simulink model "CANRXcommunication"  (R2024a)
settings: Solver=VariableStepAuto  StartTime=0.0  StopTime=10.0  RelTol=1e-3
undefined symbols (not defined in the file or in its folder): canChannel
libraries: canlib x2, canmsglib x1
settings Model: DataDictionary=BMS_System_dict1.sldd  Creator=hirah  LastModifiedBy=hirah

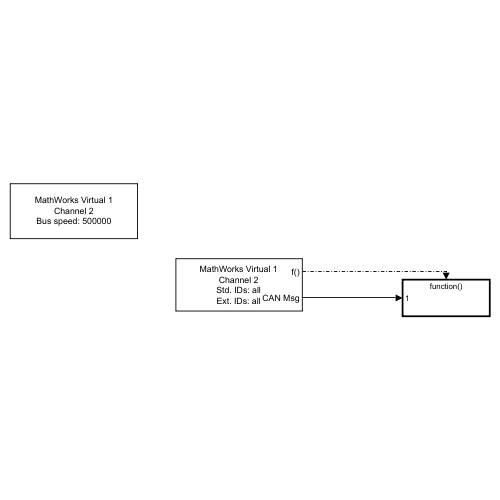
[thumbnail: Simulink's stored preview of the top-level diagram]
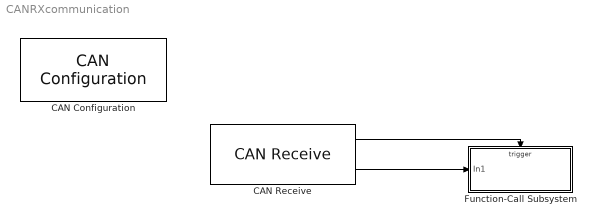
== system CANRXcommunication ==
  CAN Configuration : canlib/CAN Configuration  BlockHandle=570.0001  Device=MathWorks Virtual 1 (Channel 2)  DeviceMenu=MathWorks Virtual 1 (Channel 2)  ObjConstructor=canChannel('MathWorks', 'Virtual 1', 2)  BusSpeed=500000  EnableBitParameters=off  AckMode=Normal
  CAN Receive : canlib/CAN Receive  BlockHandle=729.0002  Device=MathWorks Virtual 1 (Channel 2)  DeviceMenu=MathWorks Virtual 1 (Channel 2)  ObjConstructor=canChannel('MathWorks', 'Virtual 1', 2)  EnableStandardIDsFilter=off  StdIDsCombo=Allow all  StandardIDs=261  EnableExtendedIDsFilter=off  ExtIDsCombo=Allow all  ExtendedIDs=0  SampleTime=0.01  MsgsPerTimestep=all  InternalFilterUpdateStatus=on  BusOutput=off
  Function-Call Subsystem : Subsystem  TreatAsAtomicUnit=on
  wires:
  CAN Receive/2 -> Function-Call Subsystem/1(In1)
  CAN Receive/1 -> Function-Call Subsystem/Trigger

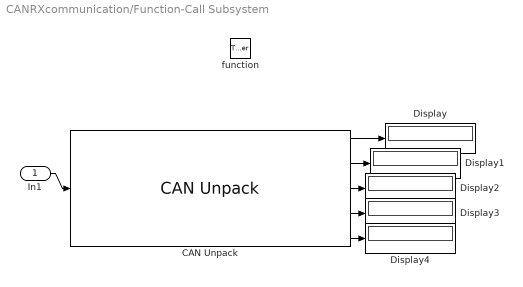
== system CANRXcommunication/Function-Call Subsystem ==
  In1 : Inport
  function : TriggerPort  TriggerType=function-call  VariantControl=(inherit)
  CAN Unpack : canmsglib/CAN Unpack  CANdbFile=C:\Users\hirah\Downloads\BMS_CAN_Database (5).dbc  MsgList=frmUDSResponse  MsgName=frmUDSResponse  MsgIDType=Standard (11-bit identifier)  MsgIdentifier=385  MsgLength=8  SignalInfo={ 'sigUDSNegativeResponseCode', '32', '8', 'LE', 'unsigned', 'Standard', '0', '1', '0', '0', '255'; 'sigUDSPositiveResponse', '0', '8', 'LE', 'unsigned', 'Standard', '0', '1', '0', '0', '255'; 'sigUDSResponseData1', '8', '8', 'LE', 'unsigned', 'Standard', '0', '1', '0', '0', '255'; 'sigUDSResponseData2', '16', '8', 'LE', 'unsigned', 'Standard', '0', '1', '0', '0', '255'; 'sigUDSResponseData3', '24', '8', 'LE', 'unsigned', 'Standard', '0', '1', '0', '0', '255' }  IDPort=off  TimestampPort=off  ErrorPort=off  RemotePort=off  LengthPort=off  StatusPort=off  ApplyMinMax=off
      settings: DataFormat=CANdb specified signals
  Display{,1..4} (5 alike) : Display
  wires:
  In1/1 -> CAN Unpack/1
  CAN Unpack/1 -> Display/1
  CAN Unpack/5 -> Display4/1
  CAN Unpack/4 -> Display3/1
  CAN Unpack/3 -> Display2/1
  CAN Unpack/2 -> Display1/1
